simulink model "digillat"  (R2024b)
settings: Solver=VariableStepAuto  StartTime=0.0  StopTime=10.0  RelTol=1e-3
settings Model: Creator=Shreesha Kumar  LastModifiedBy=Shreesha Kumar

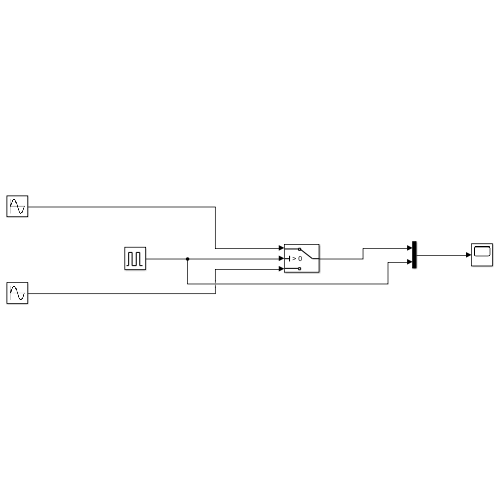
[thumbnail: Simulink's stored preview of the top-level diagram]
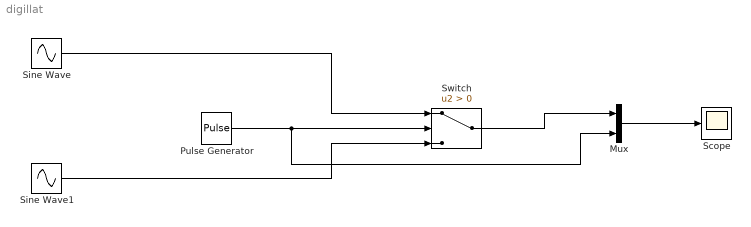
== system digillat ==
  Mux : Mux  Inputs=2
  Pulse Generator : DiscretePulseGenerator  PulseType=Time based  Period=10  PulseWidth=5
  Scope : Scope
  Sine Wave : Sin  SampleTime=0
  Sine Wave1 : Sin  SampleTime=0
  Switch : Switch  Criteria=u2 > Threshold  SaturateOnIntegerOverflow=off  InputSameDT=off
  wires:
  Mux/1 -> Scope/1
  Pulse Generator/1 -> Mux/2, Switch/2
  Sine Wave/1 -> Switch/1
  Sine Wave1/1 -> Switch/3
  Switch/1 -> Mux/1
